simulink model "Driver2_1DAC_2ADC"  (R2021a)
settings: Solver=VariableStepAuto  StartTime=0.0  StopTime=2.0e-3  RelTol=1e-3
libraries: XyceBlocks x1
settings Model: Creator=rlschie  LastModifiedBy=rlschie

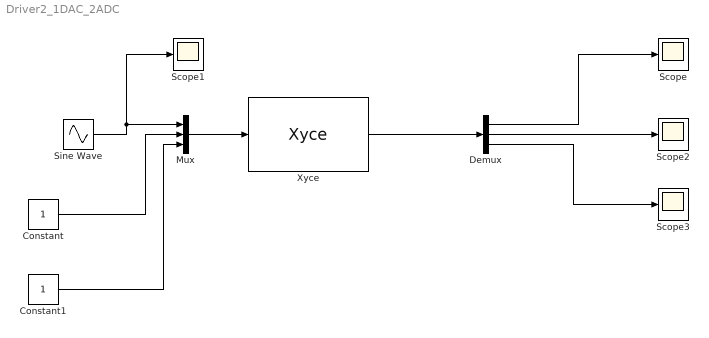
== system Driver2_1DAC_2ADC ==
  Constant : Constant
  Constant1 : Constant
  Demux : Demux  Outputs=3
  Mux : Mux  Inputs=3
  Scope{,1..3} (4 alike) : Scope
  Sine Wave : Sin  Frequency=3000  SampleTime=0
  Xyce : XyceBlocks/Xyce  UserSelectedXyceInputFileName=1Dac2ADCSystem.cir  InputNames=YDAC!DAC_DRIVER1  OutputNames=YADC!ADC1,V(N4),N(YMEMRISTOR!MR1:R)
  wires:
  Sine Wave/1 -> Mux/1, Scope1/1
  Xyce/1 -> Demux/1
  Demux/1 -> Scope/1
  Demux/2 -> Scope2/1
  Demux/3 -> Scope3/1
  Mux/1 -> Xyce/1
  Constant/1 -> Mux/2
  Constant1/1 -> Mux/3
